simulink library "ControllersFcns"  (R2014b)
settings: Solver=ode45  StartTime=0.0  StopTime=10.0  RelTol=1e-3
libraries: simulink x1
settings Model: Creator=pvinnako  LastModifiedBy=pvinnako

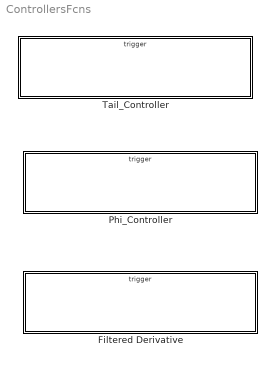
== system ControllersFcns ==
  Filtered Derivative : Subsystem  TreatAsAtomicUnit=on
  Phi_Controller : Subsystem  TreatAsAtomicUnit=on
  Tail_Controller : Subsystem  TreatAsAtomicUnit=on

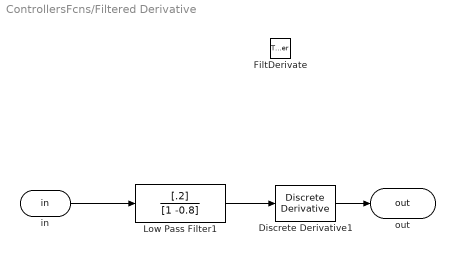
== system ControllersFcns/Filtered Derivative ==
  FiltDerivate : TriggerPort  TriggerType=function-call  IsSimulinkFunction=on  FunctionName=FiltDerivate
  Discrete Derivative1 : simulink/Discrete/Discrete Derivative  gainval=1.0  ICPrevScaledInput=0.0  InputProcessing=Inherited  OutMin=[]  OutMax=[]  OutDataType=fixdt(1, 16)  OutScaling=2^-10  DoSatur=off
  Low Pass Filter1 : DiscreteFilter  Numerator=[.2]  Denominator=[1 -0.8]
  in : ArgIn  ArgumentName=in
  out : ArgOut  ArgumentName=out
  wires:
  in/1 -> Low Pass Filter1/1
  Low Pass Filter1/1 -> Discrete Derivative1/1
  Discrete Derivative1/1 -> out/1

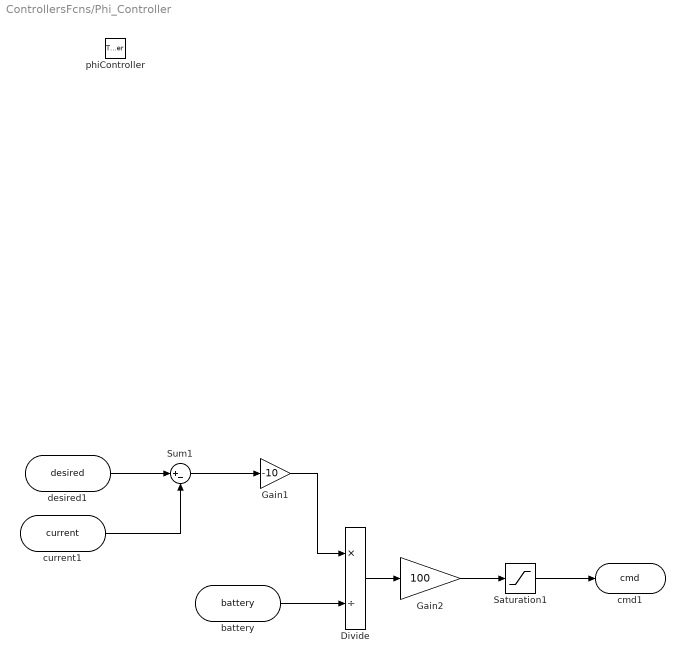
== system ControllersFcns/Phi_Controller ==
  phiController : TriggerPort  TriggerType=function-call  IsSimulinkFunction=on  FunctionName=phiController
  Divide : Product  Inputs=*/
  Gain1 : Gain  Gain=-10
  Gain2 : Gain  Gain=100
  Saturation1 : Saturate  UpperLimit=100  LowerLimit=-100  OutDataTypeStr=single
  Sum1 : Sum  Inputs=|+-
  desired1 : ArgIn  OutDataTypeStr=single  ArgumentName=desired
  current1 : ArgIn  Port=2  OutDataTypeStr=single  ArgumentName=current
      settings: LockScale=on
  battery : ArgIn  Port=3  OutDataTypeStr=single  ArgumentName=battery
      settings: LockScale=on
  cmd1 : ArgOut  OutDataTypeStr=single  ArgumentName=cmd
  wires:
  desired1/1 -> Sum1/1
  current1/1 -> Sum1/2
  Sum1/1 -> Gain1/1
  battery/1 -> Divide/2
  Gain2/1 -> Saturation1/1
  Divide/1 -> Gain2/1
  Gain1/1 -> Divide/1
  Saturation1/1 -> cmd1/1

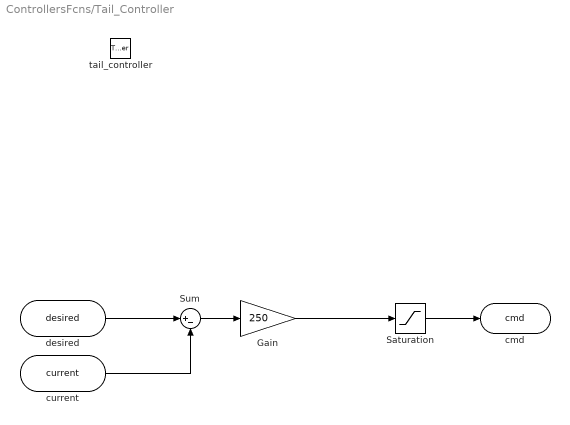
== system ControllersFcns/Tail_Controller ==
  tail_controller : TriggerPort  TriggerType=function-call  IsSimulinkFunction=on  FunctionName=tail_controller
  Gain : Gain  Gain=250
  Saturation : Saturate  UpperLimit=100  LowerLimit=-100  OutDataTypeStr=single
  Sum : Sum  Inputs=|+-
  current : ArgIn  OutDataTypeStr=single  ArgumentName=current
      settings: LockScale=on
  desired : ArgIn  Port=2  OutDataTypeStr=single  ArgumentName=desired
  cmd : ArgOut  OutDataTypeStr=single  ArgumentName=cmd
  wires:
  Saturation/1 -> cmd/1
  Gain/1 -> Saturation/1
  desired/1 -> Sum/1
  current/1 -> Sum/2
  Sum/1 -> Gain/1
